simulink model "resisti"  (R2024a)
settings: Solver=VariableStepAuto  StartTime=0.0  StopTime=10.0  RelTol=1e-3
libraries: simulink x1
settings Model: Creator=emanuele  LastModifiedBy=emanuele

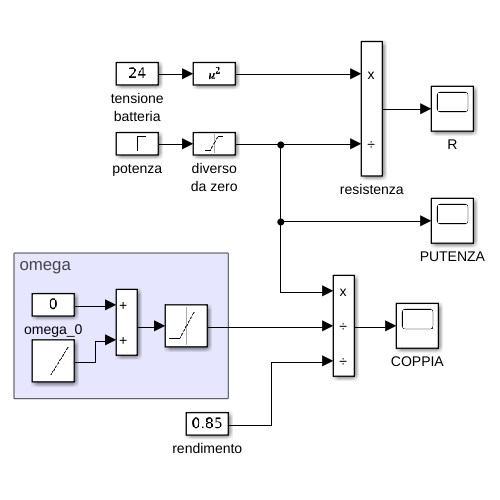
[thumbnail: Simulink's stored preview of the top-level diagram]
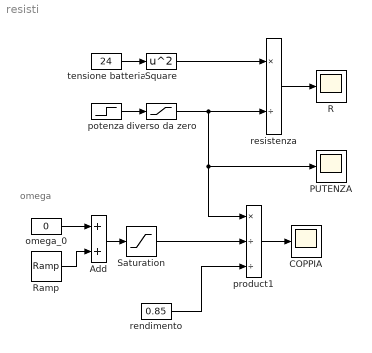
== system resisti ==
  note: omega
  Add : Sum
  COPPIA : Scope
  PUTENZA : Scope
  R : Scope
  Ramp : simulink/Sources/Ramp  slope=20  start=2  InitialOutput=0
  Saturation : Saturate  UpperLimit=180  LowerLimit=1
  Square : Math  Operator=square
  diverso da zero : Saturate  UpperLimit=10e4  LowerLimit=10e-3
  omega_0 : Constant  Value=0
  potenza : Step  Time=5  After=576  SampleTime=0
  product1 : Product  Inputs=*//
  rendimento : Constant  Value=0.85
  resistenza : Product  Inputs=*/
  tensione batteria : Constant  Value=24
  wires:
  tensione batteria/1 -> Square/1
  potenza/1 -> diverso da zero/1
  Square/1 -> resistenza/1
  diverso da zero/1 -> product1/1, PUTENZA/1, resistenza/2
  resistenza/1 -> R/1
  omega_0/1 -> Add/1
  Add/1 -> Saturation/1
  Ramp/1 -> Add/2
  Saturation/1 -> product1/2
  rendimento/1 -> product1/3
  product1/1 -> COPPIA/1
